simulink model "orbit"  (R2020b)
settings: Solver=VariableStepAuto  StartTime=0.0  StopTime=10.0  RelTol=1e-3
values from neighbouring files (symbols this model uses):
  r0_I = A_FI*rF    [main.m]
  rEarth = 6.378137e6    (= 6378137)    [main.m]
  v0_I = A_FI*vF    [main.m]
undefined symbols (not defined in the file or in its folder): IAU, WMM2020
libraries: aerolibtransform2 x2, aerolibgravity2 x2, aerolibconvert2 x1
settings Model: Creator=tjones  LastModifiedBy=tjones

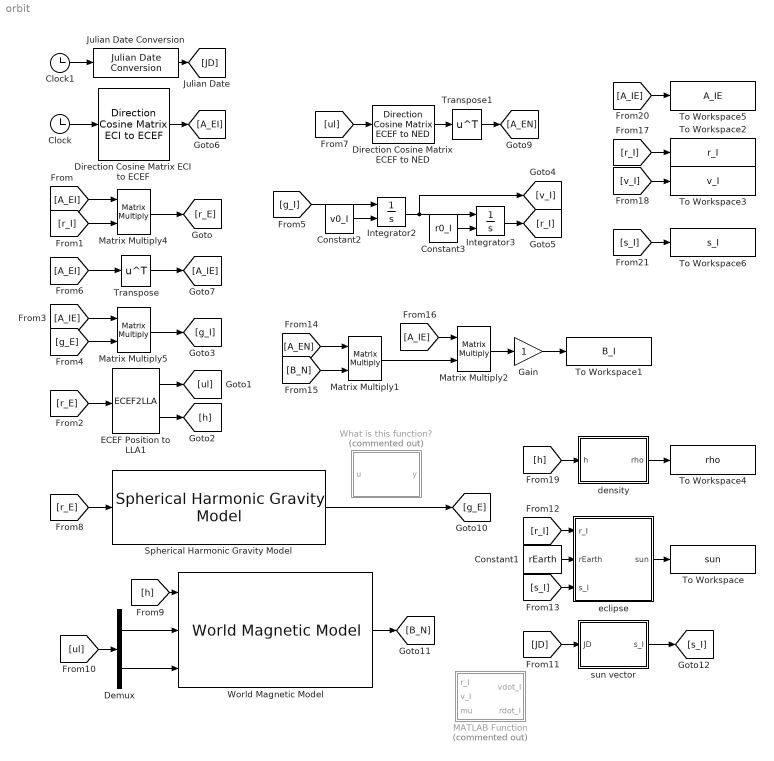
== system orbit ==
  Clock : Clock
  Clock1 : Clock
  Constant1 : Constant  Value=rEarth
  Constant2 : Constant  Value=v0_I
  Constant3 : Constant  Value=r0_I
  Demux : Demux  Outputs=2
  Direction Cosine Matrix ECEF to NED : aerolibtransform2/Direction Cosine Matrix ECEF to NED
      settings: SourceProductBaseCode=AE
  Direction Cosine Matrix ECI to ECEF : aerolibtransform2/Direction Cosine Matrix ECI to ECEF  red=IAU-2000/2006  year=2021  month=January  day=25  hour=8  min=56  sec=37  deltaT=Sec  errorflag=Error  extraparamflag=off
      settings: AttributesFormatString=%<red>  SourceProductBaseCode=AE
  ECEF Position to LLA1 : ECEF2LLA  R=6378137
  Gain : Gain
  Integrator2 : Integrator  InitialConditionSource=external
  Integrator3 : Integrator  InitialConditionSource=external
  Julian Date Conversion : aerolibconvert2/Julian Date Conversion  year=2021  month=January  day=25  hour=0  min=0  sec=0  modflag=off  deltaT=Sec  errorflag=Error
      settings: SourceProductBaseCode=AE
  MATLAB Function : MATLAB Function  Commented=on  TreatAsAtomicUnit=on
  Matrix Multiply{1..2,4..5} (4 alike) : Product  Multiplication=Matrix(*)
  Spherical Harmonic Gravity Model : aerolibgravity2/Spherical Harmonic Gravity Model  units=Metric (MKS)  degree=21  action=Warning  ptype=EGM2008  datafile='aerogmm2b.mat'
      settings: SourceProductBaseCode=AE
  To Workspace : ToWorkspace  VariableName=sun  SaveFormat=Timeseries  SampleTime=-1
  To Workspace1 : ToWorkspace  VariableName=B_I  SaveFormat=Timeseries  SampleTime=-1
  To Workspace2 : ToWorkspace  VariableName=r_I  SaveFormat=Timeseries  SampleTime=-1
  To Workspace3 : ToWorkspace  VariableName=v_I  SaveFormat=Timeseries  SampleTime=-1
  To Workspace4 : ToWorkspace  VariableName=rho  SaveFormat=Timeseries  SampleTime=-1
  To Workspace5 : ToWorkspace  VariableName=A_IE  SaveFormat=Timeseries  SampleTime=-1
  To Workspace6 : ToWorkspace  VariableName=s_I  SaveFormat=Timeseries  SampleTime=-1
  Transpose : Math  Operator=transpose  SaturateOnIntegerOverflow=on
  Transpose1 : Math  Operator=transpose  SaturateOnIntegerOverflow=on
  What is this function? : MATLAB Function  Commented=on  TreatAsAtomicUnit=on
  World Magnetic Model : aerolibgravity2/World Magnetic Model  model=WMM2020 (2020-2025)  customFile='WMM2020.COF'  units=Metric (MKS)  time_in=off  month=January  day=25  year=2021  action=Error  h_out=off  dec_out=off  inc_out=off  ti_out=off
      settings: SourceProductBaseCode=AE
  density : MATLAB Function  TreatAsAtomicUnit=on
  eclipse : MATLAB Function  TreatAsAtomicUnit=on
  sun vector : MATLAB Function  TreatAsAtomicUnit=on
  wires:
  Clock/1 -> Direction Cosine Matrix ECI to ECEF/1
  Demux/1 -> World Magnetic Model/2
  Demux/2 -> World Magnetic Model/3
  Direction Cosine Matrix ECEF to NED/1 -> Transpose1/1
  Clock1/1 -> Julian Date Conversion/1
  Matrix Multiply4/1 -> [r_E]
  [A_EI] -> Matrix Multiply4/1
  [r_I] -> Matrix Multiply4/2
  [r_E] -> ECEF Position to LLA1/1
  ECEF Position to LLA1/1 -> [ul]
  ECEF Position to LLA1/2 -> [h]
  [g_E] -> Matrix Multiply5/2
  [A_IE] -> Matrix Multiply5/1
  Matrix Multiply5/1 -> [g_I]
  Integrator2/1 -> [v_I], Integrator3/1
  Constant3/1 -> Integrator3/2
  Constant2/1 -> Integrator2/2
  [g_I] -> Integrator2/1
  Integrator3/1 -> [r_I]
  Direction Cosine Matrix ECI to ECEF/1 -> [A_EI]
  [A_EI] -> Transpose/1
  Transpose/1 -> [A_IE]
  Julian Date Conversion/1 -> [JD]
  [ul] -> Direction Cosine Matrix ECEF to NED/1
  Transpose1/1 -> [A_EN]
  [r_E] -> Spherical Harmonic Gravity Model/1
  [h] -> World Magnetic Model/1
  [ul] -> Demux/1
  World Magnetic Model/1 -> [B_N]
  [JD] -> sun vector/1(JD)
  sun vector/1(s_I) -> [s_I]
  [r_I] -> eclipse/1(r_I)
  Constant1/1 -> eclipse/2(rEarth)
  [s_I] -> eclipse/3(s_I)
  eclipse/1(sun) -> To Workspace/1
  [B_N] -> Matrix Multiply1/2
  [A_EN] -> Matrix Multiply1/1
  [A_IE] -> Matrix Multiply2/1
  Matrix Multiply1/1 -> Matrix Multiply2/2
  Matrix Multiply2/1 -> Gain/1
  Gain/1 -> To Workspace1/1
  [r_I] -> To Workspace2/1
  [v_I] -> To Workspace3/1
  [h] -> density/1(h)
  density/1(rho) -> To Workspace4/1
  [A_IE] -> To Workspace5/1
  [s_I] -> To Workspace6/1
  Spherical Harmonic Gravity Model/1 -> [g_E]

== matlab function orbit/What is this function? ==
  data: u input; y output
function y = fcn(u)

y = u;

== matlab function orbit/MATLAB Function ==
  data: r_I input; vdot_I output; v_I input; mu input; rdot_I output
function [vdot_I, rdot_I] = fcn(r_I, v_I, mu)


rdot_I = 0;
vdot_I = 0;
end

== matlab function orbit/sun vector ==
  data: JD input; s_I output
function s_I = fcn(JD)

s_I = JD;

== matlab function orbit/eclipse ==
  data: r_I input; sun output; rEarth input; s_I input
function sun = fcn(r_I, rEarth, s_I)

sun = 0;

== matlab function orbit/density ==
  data: h input; rho output
function rho = fcn(h)

rho = 0;
